simulink model "oddOReven"  (R2021a)
settings: Solver=FixedStepDiscrete  StartTime=0.0  StopTime=10.0  RelTol=1e-3  EnableMultiTasking=on
settings Model: Creator=Noha  LastModifiedBy=Noha
settings DataIOCC: ReturnWorkspaceOutputs=off
settings OptimizationCC: DefaultParameterBehavior=Inlined  InlineInvariantSignals=on  LifeSpan=1  OptimizationLevel=level1  OptimizationCustomize=off  EfficientTunableParamExpr=on
settings DebuggingCC: UnderspecifiedInitializationDetection=Classic  MergeDetectMultiDrivingBlocksExec=none  SFMachineParentedDataDiag=warning  ArithmeticOperatorsInVariantConditions=warning
settings ModelReferenceCC: PropagateSignalLabelsOutOfModel=off
settings SFSimCC: MATLABDynamicMemAlloc=off  CustomCodeUndefinedFunction=UseInterfaceOnly
settings RTWCC: SystemTargetFile=ert.tlc  GenCodeOnly=on  TemplateMakefile=ert_default_tmf  GenerateReport=on  IncludeHyperlinkInReport=on  LaunchReport=on  GenerateTraceInfo=on  GenerateTraceReport=on  GenerateTraceReportSl=on  GenerateTraceReportSf=on  GenerateTraceReportEml=on
settings CodeAppCC: ForceParamTrailComments=on  IgnoreCustomStorageClasses=off  OperatorAnnotations=on  SimulinkDataObjDesc=on  SFDataObjDesc=on  MATLABFcnDesc=on  InsertBlockDesc=on  StateflowObjectComments=on  MATLABSourceComments=on
settings ERTTargetCC: MultiwordLength=2048  GenerateSampleERTMain=on  InlinedParameterPlacement=NonHierarchical  ERTCustomFileTemplate=example_file_process.tlc

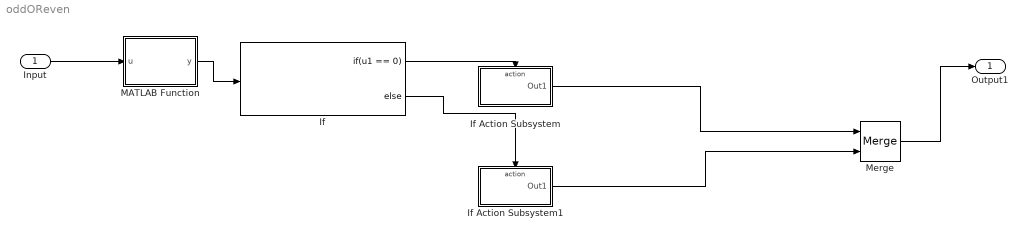
== system oddOReven ==
  Input : Inport  OutDataTypeStr=uint8
  If : If  IfExpression=u1 == 0
  If Action Subsystem : Subsystem  TreatAsAtomicUnit=on
  If Action Subsystem1 : Subsystem  TreatAsAtomicUnit=on
  MATLAB Function : MATLAB Function  TreatAsAtomicUnit=on
  Merge : Merge
  Output1 : Outport
  wires:
  MATLAB Function/1(y) -> If/1
  Input/1 -> MATLAB Function/1(u)
  Merge/1 -> Output1/1
  If/1 -> If Action Subsystem/Action
  If/2 -> If Action Subsystem1/Action
  If Action Subsystem/1(Out1) -> Merge/1
  If Action Subsystem1/1(Out1) -> Merge/2

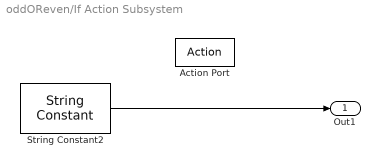
== system oddOReven/If Action Subsystem ==
  Action Port : ActionPort  ActionPortLabel=if(u1 == 0)
  String Constant2 : StringConstant  String="\"even\""
  Out1 : Outport
  wires:
  String Constant2/1 -> Out1/1

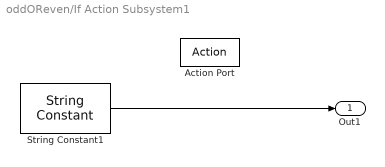
== system oddOReven/If Action Subsystem1 ==
  Action Port : ActionPort  ActionPortLabel=else
  String Constant1 : StringConstant  String="\"odd\""
  Out1 : Outport
  wires:
  String Constant1/1 -> Out1/1

== matlab function oddOReven/MATLAB Function ==
  data: u input; y output
function y = fcn(u)

y = mod(u,2);
